simulink model "following_model"  (R2021a)
settings: Solver=VariableStepAuto  StartTime=0.0  StopTime=100  RelTol=1e-3
libraries: simulink x2, vrlib x2, mpcadaslib x1
settings Model: Creator=muzaf  LastModifiedBy=muzaf

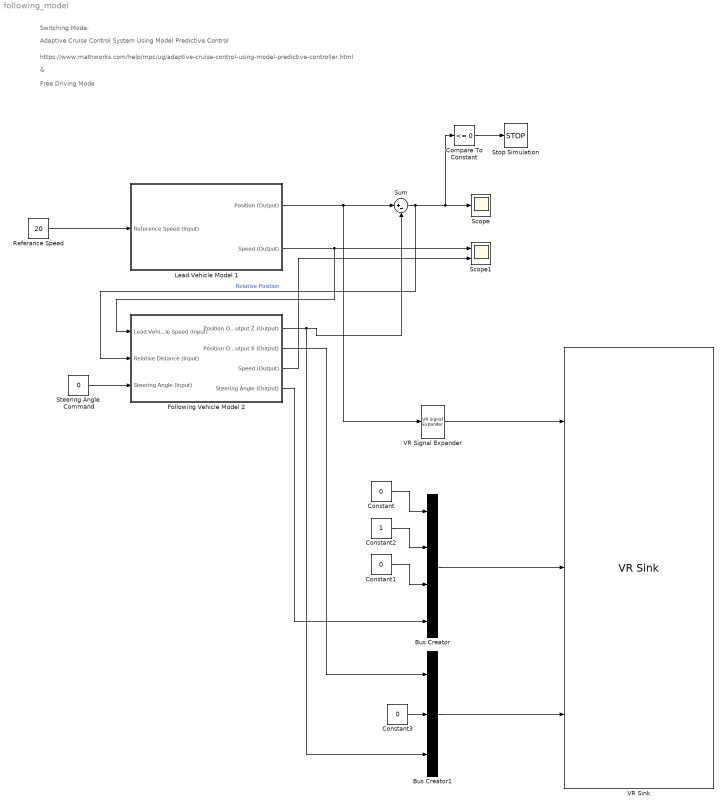
== system following_model ==
  note: Adaptive Cruise Control System Using Model Predictive Control
  note: https://www.mathworks.com/help/mpc/ug/adaptive-cruise-control-using-model-predictive-controller.html
  note: Switching Mode:
  note: &
  note: Free Driving Mode
  Bus Creator : BusCreator  Inputs=4
  Bus Creator1 : BusCreator  Inputs=3
  Compare To Constant : simulink/Logic and Bit Operations/Compare To Constant  relop=<=  const=0  OutDataTypeStr=boolean
  Constant : Constant  Value=0
  Constant1 : Constant  Value=0
  Constant2 : Constant
  Constant3 : Constant  Value=0
  Following Vehicle Model 2 : Subsystem  mask{Pos=0, Speed=25}
      mask prompts: Pos "Initial Position"; Speed "Initial Speed"
      mask TypeOptions Pos:
      | Initial Position
      | (Constant)/Value
      mask TypeOptions Speed:
      | Initial Speed
      | (Constant)/Value
  Lead Vehicle Model 1 : Subsystem  mask{Pos=35, Speed=15}
      mask prompts: Pos "Initial Position"; Speed "Initial Speed"
      mask TypeOptions Pos:
      | Initial Position
      | (Constant)/Value
      mask TypeOptions Speed:
      | Initial Speed
      | (Constant)/Value
  Referance Speed : Constant  Value=20
  Scope : Scope
  Scope1 : Scope  NumInputPorts=2
  Steering Angle Command : Constant  Value=0
  Stop Simulation : Stop
  Sum : Sum  Inputs=|+-
  VR Signal Expander : vrlib/VR Signal Expander  outwidth=3  outidx=[3]
  VR Sink : vrlib/VR Sink  InstantiateOnLoad=on  SampleTime=0.02  ViewEnable=on  RemoteChange=off  RemoteView=off  FieldsWritten=Car_Red.translation.3.1.1.double#Car_Blue.rotation.4.1.1.double#Car_Blue.translation.3.1.1.double  WorldFileName=PlatoonWorld.WRL  AutoView=off  VideoDimensions=[]  AllowVariableSize=off
  wires:
  Lead Vehicle Model 1/1(Position (Output)) -> VR Signal Expander/1, Sum/1
  Referance Speed/1 -> Lead Vehicle Model 1/1(Reference Speed (Input))
  Following Vehicle Model 2/3(Speed (Output)) -> Scope1/2
  Lead Vehicle Model 1/2(Speed (Output)) -> Following Vehicle Model 2/1(Lead Vehicle Speed (Input)), Scope1/1
  Sum/1 -> Compare To Constant/1, Scope/1, Following Vehicle Model 2/2(Relative Distance (Input))  "Relative Position"
  Compare To Constant/1 -> Stop Simulation/1
  Following Vehicle Model 2/1(Position Output Z (Output)) -> Sum/2, Bus Creator1/3
  Steering Angle Command/1 -> Following Vehicle Model 2/3(Steering Angle (Input))
  VR Signal Expander/1 -> VR Sink/1
  Following Vehicle Model 2/4(Steering Angle (Output)) -> Bus Creator/4
  Constant/1 -> Bus Creator/1
  Constant1/1 -> Bus Creator/3
  Constant2/1 -> Bus Creator/2
  Bus Creator/1 -> VR Sink/2
  Constant3/1 -> Bus Creator1/2
  Bus Creator1/1 -> VR Sink/3
  Following Vehicle Model 2/2(Position Output X (Output)) -> Bus Creator1/1

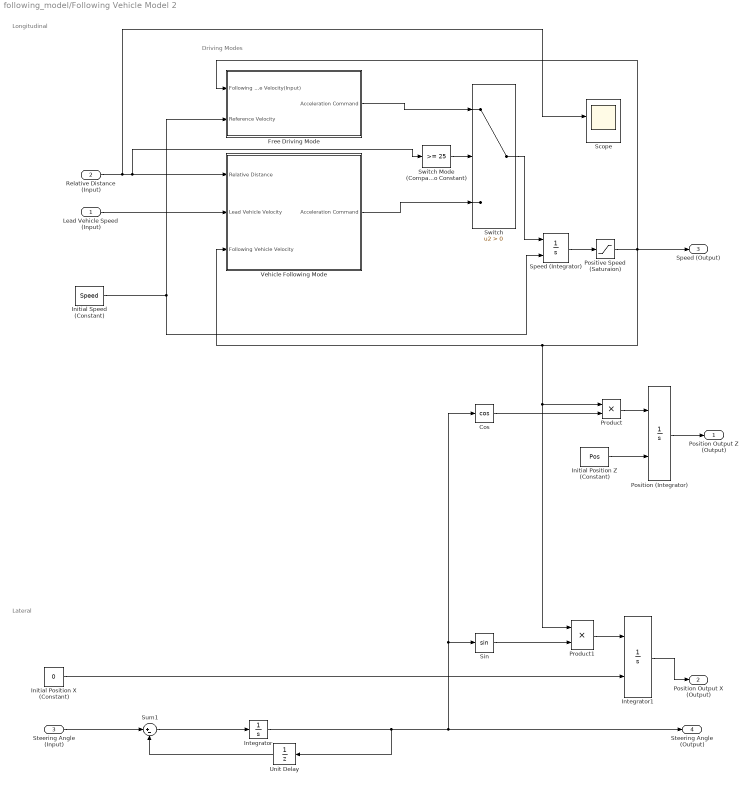
== system following_model/Following Vehicle Model 2 ==
  note: Driving Modes
  note: Lateral
  note: Longitudinal
  Lead Vehicle Speed (Input) : Inport
  Relative Distance (Input) : Inport  Port=2
  Steering Angle (Input) : Inport  Port=3
  Cos : Trigonometry  Operator=cos
  Free Driving Mode : Subsystem
  Initial Position X (Constant) : Constant  Value=0
  Initial Position Z (Constant) : Constant  Value=Pos
  Initial Speed (Constant) : Constant  Value=Speed
  Integrator : Integrator
  Integrator1 : Integrator  InitialConditionSource=external
  Position (Integrator) : Integrator  InitialConditionSource=external
  Positive Speed (Saturaion) : Saturate  UpperLimit=inf  LowerLimit=0
  Product : Product
  Product1 : Product
  Scope : Scope  NumInputPorts=4
  Sin : Trigonometry
  Speed (Integrator) : Integrator  InitialConditionSource=external
  Sum1 : Sum  Inputs=|+-
  Switch : Switch  Criteria=u2 > Threshold
  Switch Mode (Compare To Constant) : simulink/Logic and Bit Operations/Compare To Constant  relop=>=  const=25  OutDataTypeStr=boolean
  Unit Delay : UnitDelay  SampleTime=-1  HasFrameUpgradeWarning=on
  Vehicle Following Mode : Subsystem
  Position Output Z (Output) : Outport
  Position Output X (Output) : Outport  Port=2
  Speed (Output) : Outport  Port=3
  Steering Angle (Output) : Outport  Port=4
  wires:
  Initial Speed (Constant)/1 -> Free Driving Mode/2(Reference Velocity), Speed (Integrator)/2
  Speed (Integrator)/1 -> Positive Speed (Saturaion)/1
  Initial Position Z (Constant)/1 -> Position (Integrator)/2
  Positive Speed (Saturaion)/1 -> Product1/1, Product/1, Vehicle Following Mode/3(Following Vehicle Velocity), Speed (Output)/1, Free Driving Mode/1(Following Vehicle Velocity(Input))
  Position (Integrator)/1 -> Position Output Z (Output)/1
  Steering Angle (Input)/1 -> Sum1/1
  Sum1/1 -> Integrator/1
  Integrator/1 -> Unit Delay/1, Steering Angle (Output)/1, Sin/1, Cos/1
  Unit Delay/1 -> Sum1/2
  Initial Position X (Constant)/1 -> Integrator1/2
  Cos/1 -> Product/2
  Product/1 -> Position (Integrator)/1
  Sin/1 -> Product1/2
  Product1/1 -> Integrator1/1
  Integrator1/1 -> Position Output X (Output)/1
  Relative Distance (Input)/1 -> Scope/2, Switch Mode (Compare To Constant)/1, Vehicle Following Mode/1(Relative Distance)
  Lead Vehicle Speed (Input)/1 -> Vehicle Following Mode/2(Lead Vehicle Velocity)
  Vehicle Following Mode/1(Acceleration Command) -> Switch/3
  Switch/1 -> Speed (Integrator)/1
  Free Driving Mode/1(Acceleration Command) -> Switch/1
  Switch Mode (Compare To Constant)/1 -> Switch/2

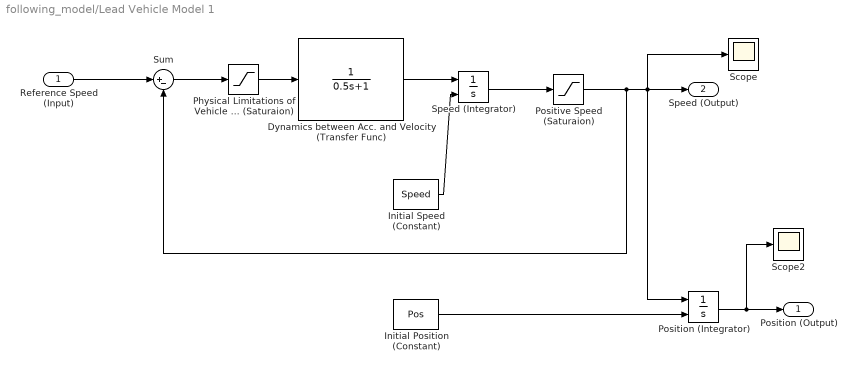
== system following_model/Lead Vehicle Model 1 ==
  Reference Speed (Input) : Inport
  Dynamics between Acc. and Velocity (Transfer Func) : TransferFcn  Denominator=[0.5 1]
  Initial Position (Constant) : Constant  Value=Pos
  Initial Speed (Constant) : Constant  Value=Speed
  Physical Limitations of Vehicle Dynamics Acceleration (Saturaion) : Saturate  UpperLimit=2  LowerLimit=-3
  Position (Integrator) : Integrator  InitialConditionSource=external
  Positive Speed (Saturaion) : Saturate  UpperLimit=inf  LowerLimit=0
  Scope : Scope
  Scope2 : Scope
  Speed (Integrator) : Integrator  InitialConditionSource=external
  Sum : Sum  Inputs=|+-
  Position (Output) : Outport
  Speed (Output) : Outport  Port=2
  wires:
  Physical Limitations of Vehicle Dynamics Acceleration (Saturaion)/1 -> Dynamics between Acc. and Velocity (Transfer Func)/1
  Reference Speed (Input)/1 -> Sum/1
  Position (Integrator)/1 -> Position (Output)/1, Scope2/1
  Dynamics between Acc. and Velocity (Transfer Func)/1 -> Speed (Integrator)/1
  Positive Speed (Saturaion)/1 -> Sum/2, Speed (Output)/1, Position (Integrator)/1, Scope/1
  Initial Position (Constant)/1 -> Position (Integrator)/2
  Sum/1 -> Physical Limitations of Vehicle Dynamics Acceleration (Saturaion)/1
  Speed (Integrator)/1 -> Positive Speed (Saturaion)/1
  Initial Speed (Constant)/1 -> Speed (Integrator)/2

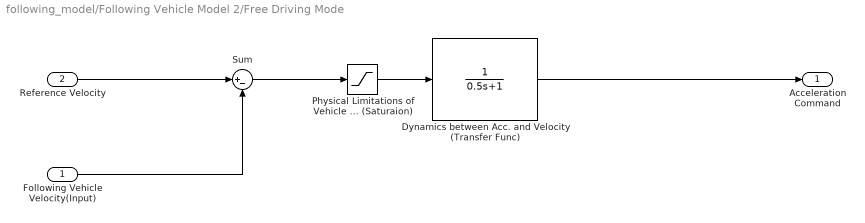
== system following_model/Following Vehicle Model 2/Free Driving Mode ==
  Following Vehicle Velocity(Input) : Inport
  Reference Velocity : Inport  Port=2
  Dynamics between Acc. and Velocity (Transfer Func) : TransferFcn  Denominator=[0.5 1]
  Physical Limitations of Vehicle Dynamics Acceleration (Saturaion) : Saturate  UpperLimit=2  LowerLimit=-3
  Sum : Sum  Inputs=|+-
  Acceleration Command : Outport
  wires:
  Reference Velocity/1 -> Sum/1
  Dynamics between Acc. and Velocity (Transfer Func)/1 -> Acceleration Command/1
  Sum/1 -> Physical Limitations of Vehicle Dynamics Acceleration (Saturaion)/1
  Physical Limitations of Vehicle Dynamics Acceleration (Saturaion)/1 -> Dynamics between Acc. and Velocity (Transfer Func)/1
  Following Vehicle Velocity(Input)/1 -> Sum/2

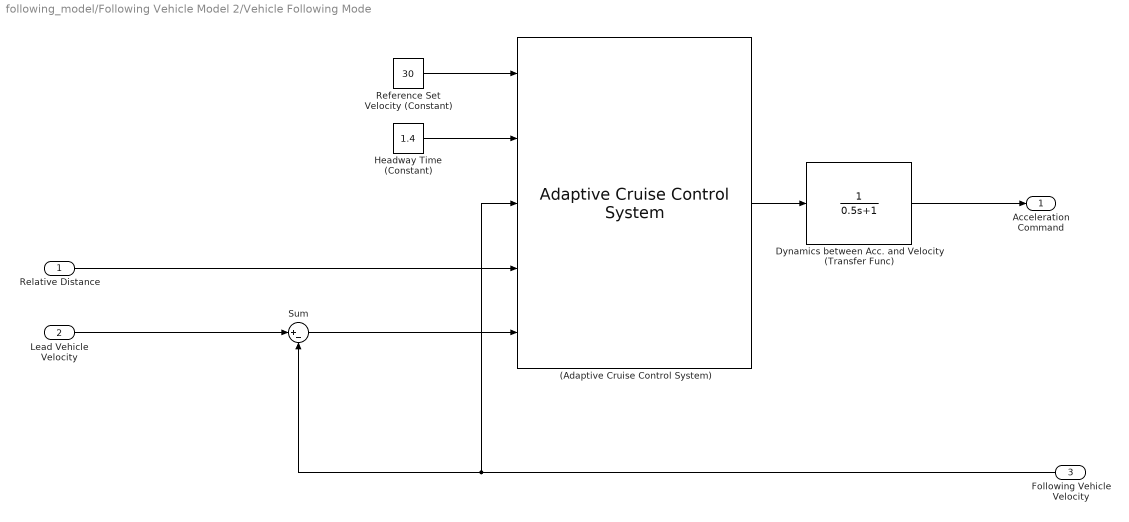
== system following_model/Following Vehicle Model 2/Vehicle Following Mode ==
  Relative Distance : Inport
  Lead Vehicle Velocity : Inport  Port=2
  Following Vehicle Velocity : Inport  Port=3
  (Adaptive Cruise Control System) : mpcadaslib/Adaptive Cruise Control System  EgoModel=tf(1,[0.5,1,0])  InitialEgoVelocity=30  DefaultSpacing=5  MaxVelocity=50  MinAcceleration=-3  amin_ext=off  MaxAcceleration=2  amax_ext=off  Ts=0.5  PredictionHorizon=200  ControllerBehavior=0.8  suboptimal=off  maxiter=10  datatypeopt=double  optmode=off  trackmode=off
  Dynamics between Acc. and Velocity (Transfer Func) : TransferFcn  Denominator=[0.5 1]
  Headway Time (Constant) : Constant  Value=1.4
  Reference Set Velocity (Constant) : Constant  Value=30
  Sum : Sum  Inputs=|+-
  Acceleration Command : Outport
  wires:
  Lead Vehicle Velocity/1 -> Sum/1
  Following Vehicle Velocity/1 -> Sum/2, (Adaptive Cruise Control System)/3
  Reference Set Velocity (Constant)/1 -> (Adaptive Cruise Control System)/1
  (Adaptive Cruise Control System)/1 -> Dynamics between Acc. and Velocity (Transfer Func)/1
  Headway Time (Constant)/1 -> (Adaptive Cruise Control System)/2
  Dynamics between Acc. and Velocity (Transfer Func)/1 -> Acceleration Command/1
  Sum/1 -> (Adaptive Cruise Control System)/5
  Relative Distance/1 -> (Adaptive Cruise Control System)/4
